simulink model "Asservissement_2023a"  (R2023a)
settings: Solver=VariableStepAuto  StartTime=0.0  StopTime=100  FixedStep=1  RelTol=1e-3
undefined symbols (not defined in the file or in its folder): asserv_t3, ca, cA, cb, cB, cc, cC, cd, cD, D, gain_cmd, gain_t1, gain_t2, gain_t3, I, K1, K12, K23, Kp1, Kp2, mode, N, offset_cmd, offset_t1, offset_t2, offset_t3, P, pert_state, pert_step, R1, R12, Rp2, sample_time, T_ambiant, tau1, tau12, tau23, tau_f1, tau_f2, tau_f3, taup1, taup2
libraries: simulink_extras x3, slpidlib x1
settings Model: Creator=vingu  LastModifiedBy=victo
settings RTWCC: GPUComputeCapability=5.0

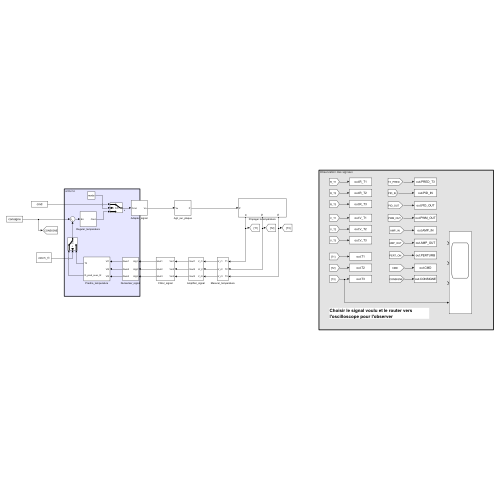
[thumbnail: Simulink's stored preview of the top-level diagram]
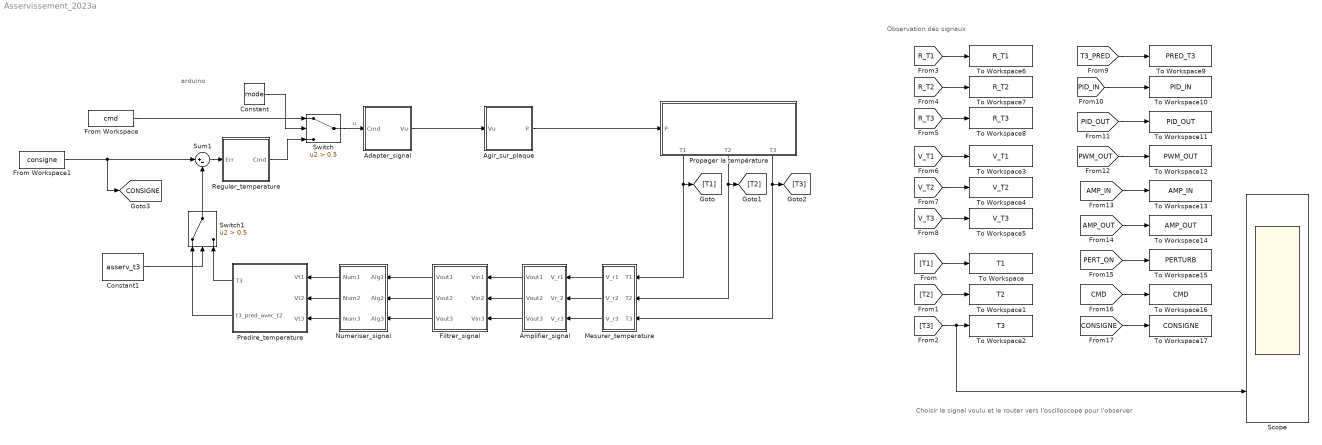
== system Asservissement_2023a ==
  note: Observation des signaux
  note: Choisir le signal voulu et le router vers l'oscilloscope pour l'observer
  note: arduino
  Adapter_signal : Subsystem
  Agir_sur_plaque : Subsystem
  Amplifier_signal : Subsystem
  Constant : Constant  Value=mode
  Constant1 : Constant  Value=asserv_t3
  Filtrer_signal : Subsystem
  From Workspace : FromWorkspace  VariableName=cmd
  From Workspace1 : FromWorkspace  VariableName=consigne
  Mesurer_temperature : Subsystem
  Numeriser_signal : Subsystem
  Predire_temperature : Subsystem
  Propager la température : Subsystem
      settings: PortSchema="{\"entries\":[{\"content\":{\"sides\":[{\"content\":{\"connectorIds\":[\"In1\"]},\"type\":\"ConnectorPlacement.EquallySpacedRectSide\",\"uuid\":\"27426f57-edaf-4249-9996-5589a3e45ee9\"},{\"content\":{\"side\":\"RIGHT\"},\"type\":\"ConnectorPlacement.EquallySpacedRectSide\",\"uuid\":\"54b45226-0e87-4404-ae6f-7d8779f7c757\"},{\"content\":{\"side\":\"TOP\"},\"type\":\"ConnectorPlacement.EquallySpacedRectSide\",\"uuid\":\"566b9fc9-30b0-40c0-87a6-76ac265a9c47\"},{\"content\":{\"connectorIds\":[\"Out1\",\"Out2\",\"Out3\"],\"side\":\"BOTTOM\"},\"type\":\"ConnectorPlacement.EquallySpacedRectSide\",\"uuid\":\"0e66943a-46b7-4cd9-83bb-3e0581ed66da\"}]},\"type\":\"ConnectorPlacement.EquallySpacedConnector\",\"uuid\":\"99e6aab4-e4b4-445a-a1ee-d65b1d9ce86f\"}],\"packageUris\":[\"http://schema.mathworks.com/mf0/Connector/R2020b\"],\"version\":\"1.0\"}"
  Reguler_temperature : Subsystem
  Scope : Scope  NumInputPorts=4
  Sum1 : Sum  Inputs=|+-
  Switch : Switch  Criteria=u2 > Threshold  Threshold=0.5  SaturateOnIntegerOverflow=off  InputSameDT=off
  Switch1 : Switch  Criteria=u2 > Threshold  Threshold=0.5  SaturateOnIntegerOverflow=off  InputSameDT=off
  To Workspace : ToWorkspace  VariableName=T1  SaveFormat=Timeseries  SampleTime=-1
  To Workspace1 : ToWorkspace  VariableName=T2  SaveFormat=Timeseries  SampleTime=-1
  To Workspace10 : ToWorkspace  VariableName=PID_IN  SaveFormat=Timeseries  SampleTime=-1
  To Workspace11 : ToWorkspace  VariableName=PID_OUT  SaveFormat=Timeseries  SampleTime=-1
  To Workspace12 : ToWorkspace  VariableName=PWM_OUT  SaveFormat=Timeseries  SampleTime=-1
  To Workspace13 : ToWorkspace  VariableName=AMP_IN  SaveFormat=Timeseries  SampleTime=-1
  To Workspace14 : ToWorkspace  VariableName=AMP_OUT  SaveFormat=Timeseries  SampleTime=-1
  To Workspace15 : ToWorkspace  VariableName=PERTURB  SaveFormat=Timeseries  SampleTime=-1
  To Workspace16 : ToWorkspace  VariableName=CMD  SaveFormat=Timeseries  SampleTime=-1
  To Workspace17 : ToWorkspace  VariableName=CONSIGNE  SaveFormat=Timeseries  SampleTime=-1
  To Workspace2 : ToWorkspace  VariableName=T3  SaveFormat=Timeseries  SampleTime=-1
  To Workspace3 : ToWorkspace  VariableName=V_T1  SaveFormat=Timeseries  SampleTime=-1
  To Workspace4 : ToWorkspace  VariableName=V_T2  SaveFormat=Timeseries  SampleTime=-1
  To Workspace5 : ToWorkspace  VariableName=V_T3  SaveFormat=Timeseries  SampleTime=-1
  To Workspace6 : ToWorkspace  VariableName=R_T1  SaveFormat=Timeseries  SampleTime=-1
  To Workspace7 : ToWorkspace  VariableName=R_T2  SaveFormat=Timeseries  SampleTime=-1
  To Workspace8 : ToWorkspace  VariableName=R_T3  SaveFormat=Timeseries  SampleTime=-1
  To Workspace9 : ToWorkspace  VariableName=PRED_T3  SaveFormat=Timeseries  SampleTime=-1
  tag scope: CONSIGNE=global
  wires:
  Amplifier_signal/1(Vout1) -> Filtrer_signal/1(Vin1)
  Amplifier_signal/2(Vout2) -> Filtrer_signal/2(Vin2)
  Sum1/1 -> Reguler_temperature/1(Err)
  Adapter_signal/1(Vu) -> Agir_sur_plaque/1(Vu)
  Mesurer_temperature/1(V_r1) -> Amplifier_signal/1(V_r1)
  Mesurer_temperature/2(V_r2) -> Amplifier_signal/2(Vr_2)
  Switch1/1 -> Sum1/2
  Filtrer_signal/3(Vout3) -> Numeriser_signal/3(Alg3)
  Mesurer_temperature/3(V_r3) -> Amplifier_signal/3(V_r3)
  Amplifier_signal/3(Vout3) -> Filtrer_signal/3(Vin3)
  Numeriser_signal/3(Num3) -> Predire_temperature/3(Vt3)
  Filtrer_signal/1(Vout1) -> Numeriser_signal/1(Alg1)
  Filtrer_signal/2(Vout2) -> Numeriser_signal/2(Alg2)
  Numeriser_signal/1(Num1) -> Predire_temperature/1(Vt1)
  Numeriser_signal/2(Num2) -> Predire_temperature/2(Vt2)
  Propager la température/3(T3) -> Mesurer_temperature/3(T3), [T3]
  From Workspace1/1 -> [CONSIGNE], Sum1/1
  Propager la température/1(T1) -> Mesurer_temperature/1(T1), [T1]
  Propager la température/2(T2) -> Mesurer_temperature/2(T2), [T2]
  Agir_sur_plaque/1(P) -> Propager la température/1(P)
  [T1] -> To Workspace/1
  [T2] -> To Workspace1/1
  [T3] -> Scope/4, To Workspace2/1
  [V_T3] -> To Workspace5/1
  [V_T2] -> To Workspace4/1
  [V_T1] -> To Workspace3/1
  [R_T3] -> To Workspace8/1
  [R_T2] -> To Workspace7/1
  [R_T1] -> To Workspace6/1
  [T3_PRED] -> To Workspace9/1
  [PID_IN] -> To Workspace10/1
  [PID_OUT] -> To Workspace11/1
  [PWM_OUT] -> To Workspace12/1
  [AMP_IN] -> To Workspace13/1
  Switch/1 -> Adapter_signal/1(Cmd)  "u"
  Constant/1 -> Switch/2
  Reguler_temperature/1(Cmd) -> Switch/3
  From Workspace/1 -> Switch/1
  [AMP_OUT] -> To Workspace14/1
  [PERT_ON] -> To Workspace15/1
  Constant1/1 -> Switch1/2
  Predire_temperature/2(t3_pred_avec_t2) -> Switch1/1
  Predire_temperature/1(T3) -> Switch1/3
  [CMD] -> To Workspace16/1
  [CONSIGNE] -> To Workspace17/1

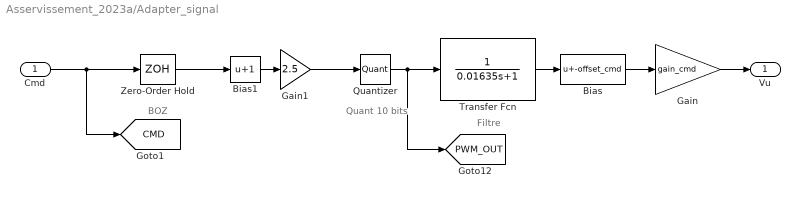
== system Asservissement_2023a/Adapter_signal ==
  note: Filtre
  note: Quant 10 bits
  note: BOZ
  Cmd : Inport
  Bias : Bias  Bias=-offset_cmd  SaturateOnIntegerOverflow=off
  Bias1 : Bias  Bias=1  SaturateOnIntegerOverflow=off
  Gain : Gain  Gain=gain_cmd
  Gain1 : Gain  Gain=2.5
  Quantizer : Quantizer  QuantizationInterval=5/(2^10-1)
  Transfer Fcn : TransferFcn  Denominator=[0.01635 1]
  Zero-Order Hold : ZeroOrderHold  SampleTime=sample_time
  Vu : Outport
  tag scope: CMD=global, PWM_OUT=global
  wires:
  Gain/1 -> Vu/1
  Transfer Fcn/1 -> Bias/1
  Bias/1 -> Gain/1
  Cmd/1 -> [CMD], Zero-Order Hold/1
  Zero-Order Hold/1 -> Bias1/1
  Gain1/1 -> Quantizer/1
  Quantizer/1 -> [PWM_OUT], Transfer Fcn/1
  Bias1/1 -> Gain1/1

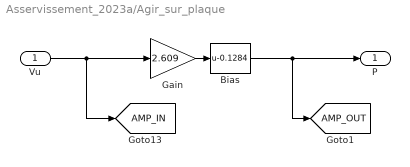
== system Asservissement_2023a/Agir_sur_plaque ==
  Vu : Inport
  Bias : Bias  Bias=-0.1284  SaturateOnIntegerOverflow=off
  Gain : Gain  Gain=2.609
  P : Outport
  tag scope: AMP_IN=global, AMP_OUT=global
  wires:
  Vu/1 -> Gain/1, [AMP_IN]
  Gain/1 -> Bias/1
  Bias/1 -> [AMP_OUT], P/1

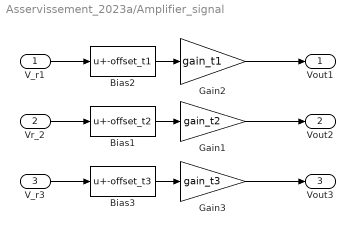
== system Asservissement_2023a/Amplifier_signal ==
  V_r1 : Inport
  Vr_2 : Inport  Port=2
  V_r3 : Inport  Port=3
  Bias1 : Bias  Bias=-offset_t2  SaturateOnIntegerOverflow=off
  Bias2 : Bias  Bias=-offset_t1  SaturateOnIntegerOverflow=off
  Bias3 : Bias  Bias=-offset_t3  SaturateOnIntegerOverflow=off
  Gain1 : Gain  Gain=gain_t2
  Gain2 : Gain  Gain=gain_t1
  Gain3 : Gain  Gain=gain_t3
  Vout1 : Outport
  Vout2 : Outport  Port=2
  Vout3 : Outport  Port=3
  wires:
  Bias1/1 -> Gain1/1
  Gain1/1 -> Vout2/1
  Vr_2/1 -> Bias1/1
  Bias2/1 -> Gain2/1
  Gain2/1 -> Vout1/1
  V_r1/1 -> Bias2/1
  V_r3/1 -> Bias3/1
  Bias3/1 -> Gain3/1
  Gain3/1 -> Vout3/1

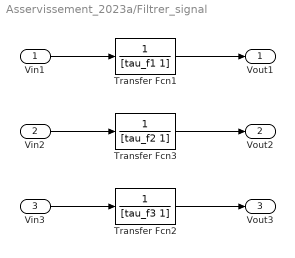
== system Asservissement_2023a/Filtrer_signal ==
  Vin1 : Inport
  Vin2 : Inport  Port=2
  Vin3 : Inport  Port=3
  Transfer Fcn1 : TransferFcn  Denominator=[tau_f1 1]
  Transfer Fcn2 : TransferFcn  Denominator=[tau_f3 1]
  Transfer Fcn3 : TransferFcn  Denominator=[tau_f2 1]
  Vout1 : Outport
  Vout2 : Outport  Port=2
  Vout3 : Outport  Port=3
  wires:
  Vin2/1 -> Transfer Fcn3/1
  Vin1/1 -> Transfer Fcn1/1
  Transfer Fcn1/1 -> Vout1/1
  Transfer Fcn3/1 -> Vout2/1
  Vin3/1 -> Transfer Fcn2/1
  Transfer Fcn2/1 -> Vout3/1

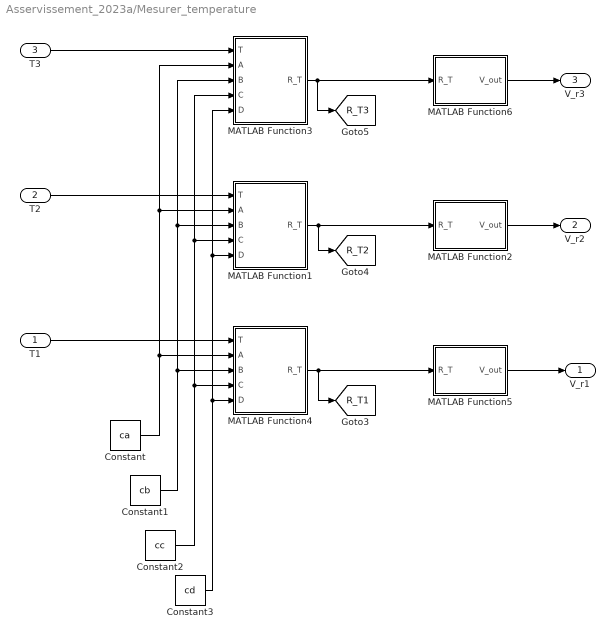
== system Asservissement_2023a/Mesurer_temperature ==
  T1 : Inport
  T2 : Inport  Port=2
  T3 : Inport  Port=3
  Constant : Constant  Value=ca
  Constant1 : Constant  Value=cb
  Constant2 : Constant  Value=cc
  Constant3 : Constant  Value=cd
  MATLAB Function1 : MATLAB Function  TreatAsAtomicUnit=on
  MATLAB Function2 : MATLAB Function  TreatAsAtomicUnit=on
  MATLAB Function3 : MATLAB Function  TreatAsAtomicUnit=on
  MATLAB Function4 : MATLAB Function  TreatAsAtomicUnit=on
  MATLAB Function5 : MATLAB Function  TreatAsAtomicUnit=on
  MATLAB Function6 : MATLAB Function  TreatAsAtomicUnit=on
  V_r1 : Outport
  V_r2 : Outport  Port=2
  V_r3 : Outport  Port=3
  tag scope: R_T1=global, R_T2=global, R_T3=global
  wires:
  MATLAB Function4/1(R_T) -> [R_T1], MATLAB Function5/1(R_T)
  MATLAB Function5/1(V_out) -> V_r1/1
  T1/1 -> MATLAB Function4/1(T)
  MATLAB Function2/1(V_out) -> V_r2/1
  MATLAB Function1/1(R_T) -> [R_T2], MATLAB Function2/1(R_T)
  T3/1 -> MATLAB Function3/1(T)
  MATLAB Function3/1(R_T) -> [R_T3], MATLAB Function6/1(R_T)
  MATLAB Function6/1(V_out) -> V_r3/1
  T2/1 -> MATLAB Function1/1(T)
  Constant3/1 -> MATLAB Function3/5(D), MATLAB Function1/5(D), MATLAB Function4/5(D)
  Constant2/1 -> MATLAB Function3/4(C), MATLAB Function1/4(C), MATLAB Function4/4(C)
  Constant1/1 -> MATLAB Function3/3(B), MATLAB Function1/3(B), MATLAB Function4/3(B)
  Constant/1 -> MATLAB Function3/2(A), MATLAB Function1/2(A), MATLAB Function4/2(A)

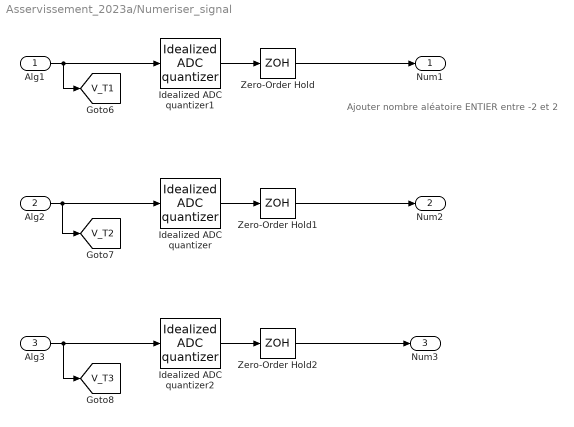
== system Asservissement_2023a/Numeriser_signal ==
  note: Ajouter nombre aléatoire ENTIER entre -2 et 2
  Alg1 : Inport
  Alg2 : Inport  Port=2
  Alg3 : Inport  Port=3
  Idealized ADC quantizer : simulink_extras/Additional Discrete/Idealized ADC quantizer  NumberOfConverterBits=bits_ADC  Vmin=0  Vmax=5  OutputDataType=int16  OutputNegativeValues=off
  Idealized ADC quantizer1 : simulink_extras/Additional Discrete/Idealized ADC quantizer  NumberOfConverterBits=bits_ADC  Vmin=0  Vmax=5  OutputDataType=int16  OutputNegativeValues=off
  Idealized ADC quantizer2 : simulink_extras/Additional Discrete/Idealized ADC quantizer  NumberOfConverterBits=bits_ADC  Vmin=0  Vmax=5  OutputDataType=int16  OutputNegativeValues=off
  Zero-Order Hold : ZeroOrderHold  SampleTime=sample_time
  Zero-Order Hold1 : ZeroOrderHold  SampleTime=sample_time
  Zero-Order Hold2 : ZeroOrderHold  SampleTime=sample_time
  Num1 : Outport
  Num2 : Outport  Port=2
  Num3 : Outport  Port=3
  tag scope: V_T1=global, V_T2=global, V_T3=global
  wires:
  Alg1/1 -> [V_T1], Idealized ADC quantizer1/1
  Alg2/1 -> [V_T2], Idealized ADC quantizer/1
  Idealized ADC quantizer1/1 -> Zero-Order Hold/1
  Idealized ADC quantizer/1 -> Zero-Order Hold1/1
  Zero-Order Hold1/1 -> Num2/1
  Zero-Order Hold/1 -> Num1/1
  Idealized ADC quantizer2/1 -> Zero-Order Hold2/1
  Zero-Order Hold2/1 -> Num3/1
  Alg3/1 -> [V_T3], Idealized ADC quantizer2/1

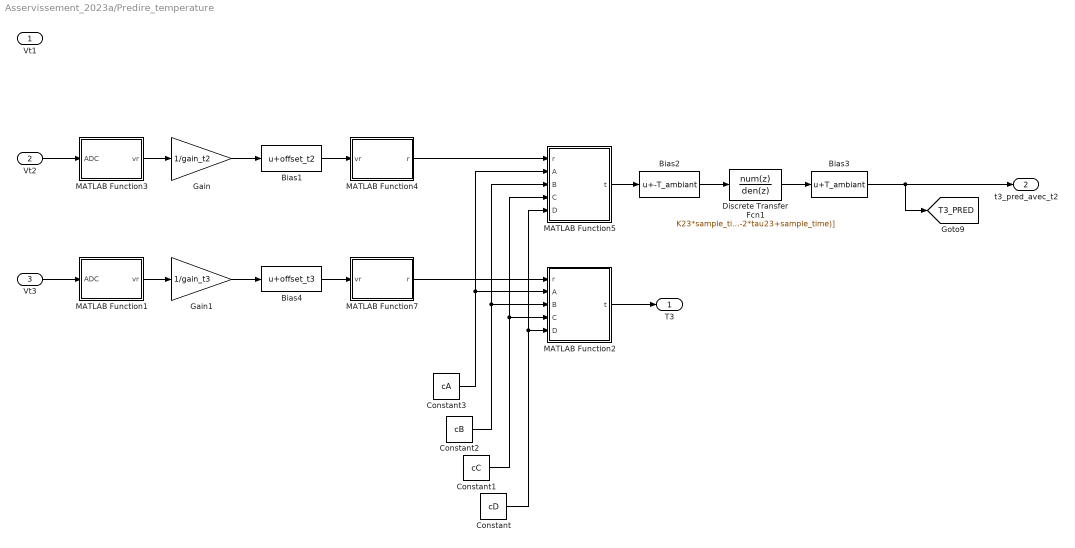
== system Asservissement_2023a/Predire_temperature ==
  Vt1 : Inport
  Vt2 : Inport  Port=2
  Vt3 : Inport  Port=3
  Bias1 : Bias  Bias=offset_t2  SaturateOnIntegerOverflow=off
  Bias2 : Bias  Bias=-T_ambiant  SaturateOnIntegerOverflow=off
  Bias3 : Bias  Bias=T_ambiant  SaturateOnIntegerOverflow=off
  Bias4 : Bias  Bias=offset_t3  SaturateOnIntegerOverflow=off
  Constant : Constant  Value=cD
  Constant1 : Constant  Value=cC
  Constant2 : Constant  Value=cB
  Constant3 : Constant  Value=cA
  Discrete Transfer Fcn1 : DiscreteTransferFcn  Numerator=K23*sample_time*[1 1]  Denominator=[(2*tau23+sample_time) (-2*tau23+sample_time)]
  Gain : Gain  Gain=1/gain_t2
  Gain1 : Gain  Gain=1/gain_t3
  MATLAB Function1 : MATLAB Function  TreatAsAtomicUnit=on
  MATLAB Function2 : MATLAB Function  TreatAsAtomicUnit=on
  MATLAB Function3 : MATLAB Function  TreatAsAtomicUnit=on
  MATLAB Function4 : MATLAB Function  TreatAsAtomicUnit=on
  MATLAB Function5 : MATLAB Function  TreatAsAtomicUnit=on
  MATLAB Function7 : MATLAB Function  TreatAsAtomicUnit=on
  T3 : Outport
  t3_pred_avec_t2 : Outport  Port=2
  tag scope: T3_PRED=global
  wires:
  MATLAB Function2/1(t) -> T3/1
  MATLAB Function4/1(r) -> MATLAB Function5/1(r)
  Vt2/1 -> MATLAB Function3/1(ADC)
  Vt3/1 -> MATLAB Function1/1(ADC)
  MATLAB Function5/1(t) -> Bias2/1
  Discrete Transfer Fcn1/1 -> Bias3/1
  Bias3/1 -> [T3_PRED], t3_pred_avec_t2/1
  Bias2/1 -> Discrete Transfer Fcn1/1
  Gain/1 -> Bias1/1
  Gain1/1 -> Bias4/1
  MATLAB Function3/1(vr) -> Gain/1
  MATLAB Function1/1(vr) -> Gain1/1
  Bias1/1 -> MATLAB Function4/1(vr)
  Bias4/1 -> MATLAB Function7/1(vr)
  MATLAB Function7/1(r) -> MATLAB Function2/1(r)
  Constant/1 -> MATLAB Function5/5(D), MATLAB Function2/5(D)
  Constant1/1 -> MATLAB Function5/4(C), MATLAB Function2/4(C)
  Constant2/1 -> MATLAB Function2/3(B), MATLAB Function5/3(B)
  Constant3/1 -> MATLAB Function5/2(A), MATLAB Function2/2(A)

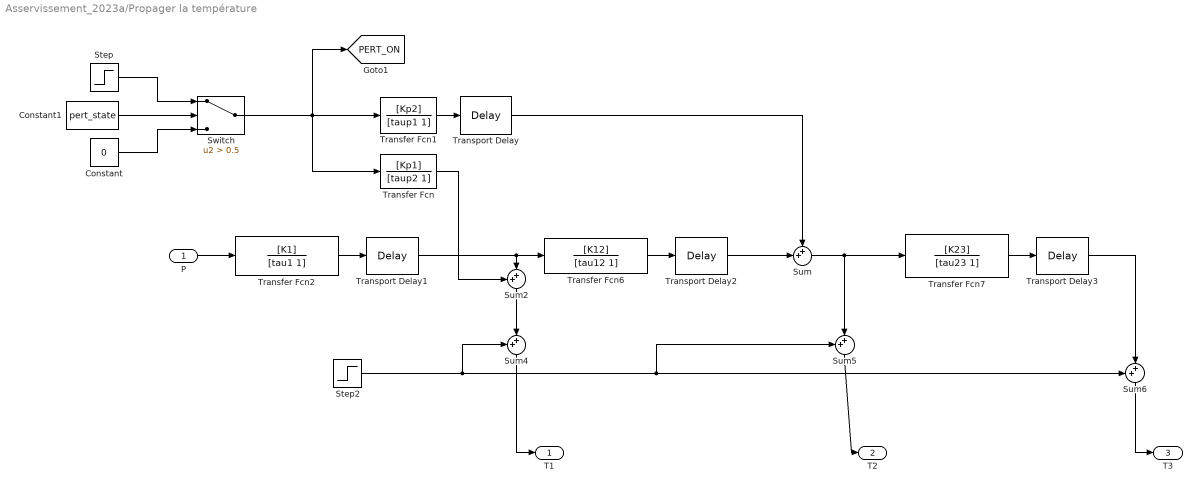
== system Asservissement_2023a/Propager la température ==
  P : Inport
  Constant : Constant  Value=0
  Constant1 : Constant  Value=pert_state
  Step : Step  Time=pert_step  SampleTime=0
  Step2 : Step  Time=-1  After=T_ambiant  SampleTime=0
  Sum{,2,4..6} (5 alike) : Sum  Inputs=++|
  Switch : Switch  Criteria=u2 > Threshold  Threshold=0.5  SaturateOnIntegerOverflow=off  InputSameDT=off
  Transfer Fcn : TransferFcn  Numerator=[Kp1]  Denominator=[taup2 1]
  Transfer Fcn1 : TransferFcn  Numerator=[Kp2]  Denominator=[taup1 1]
  Transfer Fcn2 : TransferFcn  Numerator=[K1]  Denominator=[tau1 1]
  Transfer Fcn6 : TransferFcn  Numerator=[K12]  Denominator=[tau12 1]
  Transfer Fcn7 : TransferFcn  Numerator=[K23]  Denominator=[tau23 1]
  Transport Delay : TransportDelay  DelayTime=Rp2
  Transport Delay1 : TransportDelay  DelayTime=R1
  Transport Delay2 : TransportDelay  DelayTime=R12
  Transport Delay3 : TransportDelay  DelayTime=R12
  T1 : Outport
  T2 : Outport  Port=2
  T3 : Outport  Port=3
  tag scope: PERT_ON=global
  wires:
  Sum5/1 -> T2/1
  Transport Delay/1 -> Sum/1
  Sum/1 -> Sum5/2, Transfer Fcn7/1
  Transfer Fcn1/1 -> Transport Delay/1
  P/1 -> Transfer Fcn2/1
  Step2/1 -> Sum4/1, Sum5/1, Sum6/1
  Sum2/1 -> Sum4/2
  Transfer Fcn/1 -> Sum2/1
  Sum6/1 -> T3/1
  Sum4/1 -> T1/1
  Switch/1 -> [PERT_ON], Transfer Fcn/1, Transfer Fcn1/1
  Step/1 -> Switch/1
  Constant/1 -> Switch/3
  Constant1/1 -> Switch/2
  Transfer Fcn2/1 -> Transport Delay1/1
  Transport Delay1/1 -> Sum2/2, Transfer Fcn6/1
  Transfer Fcn6/1 -> Transport Delay2/1
  Transport Delay2/1 -> Sum/2
  Transfer Fcn7/1 -> Transport Delay3/1
  Transport Delay3/1 -> Sum6/2

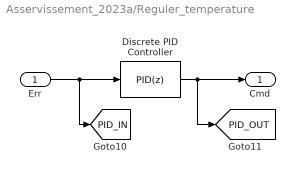
== system Asservissement_2023a/Reguler_temperature ==
  Err : Inport
  Discrete PID Controller : slpidlib/PID Controller  Controller=PID  Form=Parallel  TimeDomain=Discrete-time  UseExternalTs=off  SampleTime=sample_time  IntegratorMethod=Trapezoidal  FilterMethod=Trapezoidal  ControllerParametersSource=internal  P=P  I=I  UseKiTs=off  D=D  N=N  UseFilter=on  TunerSelectOption=Transfer Function Based (PID Tuner App)  InitialConditionSource=internal  InitialConditionForIntegrator=0  InitialConditionForFilter=0  DifferentiatorICPrevScaledInput=0  ExternalReset=none  TrackingMode=off  Kt=1  LimitOutput=on  SatLimitsSource=internal  UpperSaturationLimit=1  LowerSaturationLimit=-1  LinearizeAsGain=off  AntiWindupMode=clamping  Kb=1  LimitIntegrator=on  UpperIntegratorSaturationLimit=1  LowerIntegratorSaturationLimit=-1  POutMin=[]  POutMax=[]  IOutMin=[]  IOutMax=[]  DOutMin=[]  DOutMax=[]  NOutMin=[]  NOutMax=[]  SumOutMin=[]  SumOutMax=[]  SaturationOutMin=[]  SaturationOutMax=[]  PParamMin=[]  PParamMax=[]  IParamMin=[]  IParamMax=[]  DParamMin=[]  DParamMax=[]  NParamMin=[]  NParamMax=[]  KbParamMin=[]  KbParamMax=[]  KtParamMin=[]  KtParamMax=[]  KbOutMin=[]  KbOutMax=[]  KtOutMin=[]  KtOutMax=[]  IntegratorOutMin=[]  IntegratorOutMax=[]  FilterOutMin=[]  FilterOutMax=[]  SumI1OutMin=[]  SumI1OutMax=[]  SumI2OutMin=[]  SumI2OutMax=[]  SumI3OutMin=[]  SumI3OutMax=[]  SumI4OutMin=[]  SumI4OutMax=[]  SumDOutMin=[]  SumDOutMax=[]  DifferentiatorOutMin=[]  DifferentiatorOutMax=[]  FilterDiffOutCoefMin=[]  FilterDiffOutCoefMax=[]  ReciprocalOutMin=[]  ReciprocalOutMax=[]  SumDenOutMin=[]  SumDenOutMax=[]  SumNumOutMin=[]  SumNumOutMax=[]  DivideOutMin=[]  DivideOutMax=[]  UdiffTsProdOutMin=[]  UdiffTsProdOutMax=[]  NTsProdOutMin=[]  NTsProdOutMax=[]  UintegralTsProdOutMin=[]  UintegralTsProdOutMax=[]  UngainTsProdOutMin=[]  UngainTsProdOutMax=[]  ClampingZeroOutDataTypeStr=Inherit: Inherit via back propagation  ClampingZeroOutMin=[]  ClampingZeroOutMax=[]  FilterDenConstantOutDataTypeStr=Inherit: Inherit via back propagation  FilterDenConstantOutMin=[]  FilterDenConstantOutMax=[]  PCopyOutDataTypeStr=Inherit: Inherit via back propagation  PCopyOutMin=[]  PCopyOutMax=[]  NCopyOutDataTypeStr=Inherit: Inherit via back propagation  NCopyOutMin=[]  NCopyOutMax=[]  IntegratorContinuousStateAttributes=''  IntegratorStateMustResolveToSignalObject=off  IntegratorRTWStateStorageClass=Auto  FilterContinuousStateAttributes=''  FilterStateMustResolveToSignalObject=off  FilterRTWStateStorageClass=Auto  ParallelPVariant=InternalParameters  IdealPVariant=Disabled  IVariant=InternalParameters  DVariant=InternalParameters  IntegratorVariant=Discrete  SatVariant=Enabled  AWVariant=DiscClampingParallel  PCopyVariant=Disabled  TRVariant=Disabled  FdbkBlocksVariant=Feedback  IdealPFdbkVariant=Passthrough  SatFdbkVariant=Passthrough  DerivativeFilterVariant=TrapezoidalFilter  NVariant=InternalParameters  NCopyVariant=InternalParameters  FilterICVariant=InternalICsFilter  IntegratorICVariant=InternalICs  ExternalResetVariant=Disabled  TRSumVariant=Passthrough  SumFdbkVariant=Enabled  SumVariant=Sum_PID  TsampFilterVariant=InternalTs  TsampNgainVariant=Passthrough  TsampIntegralVariant=Disabled_SignalSpec  ExternalSaturationOutDataTypeStr=Inherit: Same as second input
      settings: LibrarySourceBlock=simulink/Discrete/Discrete PID Controller
  Cmd : Outport
  tag scope: PID_IN=global, PID_OUT=global
  wires:
  Discrete PID Controller/1 -> [PID_OUT], Cmd/1
  Err/1 -> [PID_IN], Discrete PID Controller/1

== matlab function Asservissement_2023a/Mesurer_temperature/MATLAB Function6 ==
  data: R_T input; V_out output
function V_out = calcVoltageT3(R_T)

    R_par = 820e3;
    R_serie = 10e3;
    V_in = 5;

    R_eq = (R_T * R_par) / (R_T + R_par);

    V_out = V_in * (R_eq / (R_eq + R_serie));
end

== matlab function Asservissement_2023a/Predire_temperature/MATLAB Function7 ==
  data: vr input; r output
function r = resistance3(vr)
    
    R0=10000;
    R=vr*R0/(5-vr);
    r= 820000*R/(820000-R);
end

== matlab function Asservissement_2023a/Predire_temperature/MATLAB Function1 ==
  data: ADC input; vr output
function vr = tension(ADC)

    adc = cast(ADC, "single");
    
    vr= adc*5/1024;
end

== matlab function Asservissement_2023a/Mesurer_temperature/MATLAB Function1 ==
  data: T input; R_T output; A input; B input; C input; D input
function R_T = calcResistance(T, A, B, C, D)
    
    R0 = 10000;  
    %A = -14.65719769;
    %B = 4798.842;
    %C = -115334;
    %D = -3730535;
 
    T_kelvin = T + 273.15;

    expo = A + B/T_kelvin + C/T_kelvin^2 + D/T_kelvin^3;

    R_T = R0 * exp(expo);
end

== matlab function Asservissement_2023a/Mesurer_temperature/MATLAB Function4 ==
  data: T input; R_T output; A input; B input; C input; D input
function R_T = calcResistance(T, A, B, C, D)
    
    R0 = 10000;  
    %A = -14.65719769;
    %B = 4798.842;
    %C = -115334;
    %D = -3730535;
 
    T_kelvin = T + 273.15;

    expo = A + B/T_kelvin + C/T_kelvin^2 + D/T_kelvin^3;

    R_T = R0 * exp(expo);
end

== matlab function Asservissement_2023a/Predire_temperature/MATLAB Function2 ==
  data: r input; t output; A input; B input; C input; D input
function t = temperature(r, A, B, C, D)
    
    %A = 0.00335401643468053;
    %B = 0.000256523550896126;
    %C = 0.00000260597012072052;
    %D = 0.000000063292612648746;
    R25 = 10000;
    
    t= 1/(A + B*log(r/R25) + C*log(r/R25)^2 + D*log(r/R25)^3) - 273.15;
end

== matlab function Asservissement_2023a/Mesurer_temperature/MATLAB Function5 ==
  data: R_T input; V_out output
function V_out = calcVoltageT1(R_T)

    R_par = 930e3;
    R_serie = 10e3;
    V_in = 5;

    R_eq = (R_T * R_par) / (R_T + R_par);

    V_out = V_in * (R_eq / (R_eq + R_serie));
end

== matlab function Asservissement_2023a/Mesurer_temperature/MATLAB Function2 ==
  data: R_T input; V_out output
function V_out = calcVoltageT2(R_T)

    R_par = 1380e3;
    R_serie = 10e3;
    V_in = 5;

    R_eq = (R_T * R_par) / (R_T + R_par);

    V_out = V_in * (R_eq / (R_eq + R_serie));
end

== matlab function Asservissement_2023a/Predire_temperature/MATLAB Function3 ==
  data: ADC input; vr output
function vr = tension(ADC)

    adc = cast(ADC, "single");
    
    vr= adc*5/1024;
end

== matlab function Asservissement_2023a/Predire_temperature/MATLAB Function4 ==
  data: vr input; r output
function r = resistance2(vr)
    
    R0=10000;
    R=vr*R0/(5-vr);
    r= 1380000*R/(1380000-R);
end

== matlab function Asservissement_2023a/Predire_temperature/MATLAB Function5 ==
  data: r input; t output; A input; B input; C input; D input
function t = temperature(r, A, B, C, D)
    
    %A = 0.00335401643468053;
    %B = 0.000256523550896126;
    %C = 0.00000260597012072052;
    %D = 0.000000063292612648746;
    R25 = 10000;
    
    t= 1/(A + B*log(r/R25) + C*log(r/R25)^2 + D*log(r/R25)^3) - 273.15;
end

== matlab function Asservissement_2023a/Mesurer_temperature/MATLAB Function3 ==
  data: T input; R_T output; A input; B input; C input; D input
function R_T = calcResistance(T, A, B, C, D)
    
    R0 = 10000;  
    %A = -14.65719769;
    %B = 4798.842;
    %C = -115334;
    %D = -3730535;
 
    T_kelvin = T + 273.15;

    expo = A + B/T_kelvin + C/T_kelvin^2 + D/T_kelvin^3;

    R_T = R0 * exp(expo);
end
